simulink model "quad_LQRaccControl_sim"  (R2020a)
settings: Solver=ode4  StartTime=0.0  StopTime=10  FixedStep=0.001  RelTol=1e-3
values from neighbouring files (symbols this model uses):
  L = 0.2    [anim_2Dquad.m]    (also in anim_2Dquad_intercept.m)
undefined symbols (not defined in the file or in its folder): g, I, K, m
settings Model: Creator=Amir  LastModifiedBy=alex
settings DataIOCC: ReturnWorkspaceOutputs=off
settings DebuggingCC: ArithmeticOperatorsInVariantConditions=warning
settings SFSimCC: CustomCodeUndefinedFunction=UseInterfaceOnly

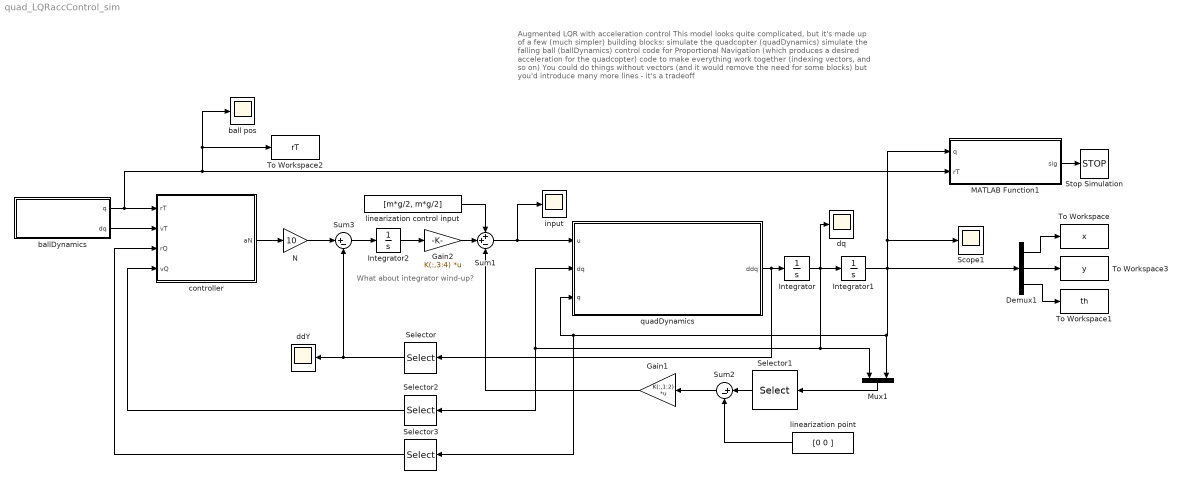
== system quad_LQRaccControl_sim ==
  note: Augmented LQR with acceleration control
      | This model looks quite complicated, but it's made up of a few (much simpler) building blocks:
      |
      | simulate the quadcopter (quadDynamics)
      | simulate the falling ball (ballDynamics)
      | control code for Proportional Navigation (which produces a desired acceleration for the quadcopter)
      | code to make everything work together (indexing vectors, and so on)
      |
      | You could do things without vectors (and it would remove the need for some blocks) but you'd introduce many more lines - it's a tradeoff
  note: What about integrator wind-up?
  Demux1 : Demux  Outputs=3
  Gain1 : Gain  Gain=K(:,1:2)  Multiplication=Matrix(K*u)
  Gain2 : Gain  Gain=K(:,3:4)  Multiplication=Matrix(K*u)
  Integrator : Integrator  InitialCondition=[0 0 0]
  Integrator1 : Integrator  InitialCondition=[0, 0, 0]
  Integrator2 : Integrator
  MATLAB Function1 : MATLAB Function  TreatAsAtomicUnit=on
  Mux1 : Mux  Inputs=2
  N : Gain  Gain=10
  Scope1 : Scope
  Selector : Selector  InputPortWidth=3  IndexOptions=Index vector (dialog)  Indices=[1 2]  OutputSizes=1
  Selector1 : Selector  InputPortWidth=6  IndexOptions=Index vector (dialog)  Indices=[3 6]  OutputSizes=1
  Selector2 : Selector  InputPortWidth=3  IndexOptions=Index vector (dialog)  Indices=[1 2]  OutputSizes=1
  Selector3 : Selector  InputPortWidth=3  IndexOptions=Index vector (dialog)  Indices=[1 2]  OutputSizes=1
  Stop Simulation : Stop
  Sum1 : Sum  Inputs=++-
  Sum2 : Sum  Inputs=|+-
  Sum3 : Sum  Inputs=|+-
  To Workspace : ToWorkspace  VariableName=x  SaveFormat=Structure With Time  SampleTime=0.01
  To Workspace1 : ToWorkspace  VariableName=th  SaveFormat=Structure With Time  SampleTime=0.01
  To Workspace2 : ToWorkspace  VariableName=rT  SaveFormat=Structure With Time  SampleTime=0.01
  To Workspace3 : ToWorkspace  VariableName=y  SaveFormat=Structure With Time  SampleTime=0.01
  ball pos : Scope
  ballDynamics : Subsystem
  controller : MATLAB Function  TreatAsAtomicUnit=on
  ddY : Scope
  dq : Scope
  input : Scope
  linearization control input : Constant  Value=[m*g/2, m*g/2]
  linearization point : Constant  Value=[0 0 ]
  quadDynamics : MATLAB Function  TreatAsAtomicUnit=on
  wires:
  quadDynamics/1(ddq) -> Integrator/1, Selector/1
  Integrator/1 -> Integrator1/1, dq/1, Mux1/1, Selector2/1, quadDynamics/2(dq)
  Sum1/1 -> input/1, quadDynamics/1(u)
  Sum2/1 -> Gain1/1
  linearization point/1 -> Sum2/2
  Integrator1/1 -> Demux1/1, Mux1/2, Selector3/1, quadDynamics/3(q), Scope1/1, MATLAB Function1/1(q)
  Demux1/3 -> To Workspace1/1
  Demux1/1 -> To Workspace/1
  Demux1/2 -> To Workspace3/1
  linearization control input/1 -> Sum1/1
  Gain1/1 -> Sum1/3
  Integrator2/1 -> Gain2/1
  Gain2/1 -> Sum1/2
  Sum3/1 -> Integrator2/1
  Selector/1 -> ddY/1, Sum3/2
  Mux1/1 -> Selector1/1
  Selector1/1 -> Sum2/1
  Selector2/1 -> controller/4(vQ)
  Selector3/1 -> controller/3(rQ)
  controller/1(aN) -> N/1
  N/1 -> Sum3/1
  MATLAB Function1/1(sig) -> Stop Simulation/1
  ballDynamics/1(q) -> MATLAB Function1/2(rT), ball pos/1, To Workspace2/1, controller/1(rT)
  ballDynamics/2(dq) -> controller/2(vT)

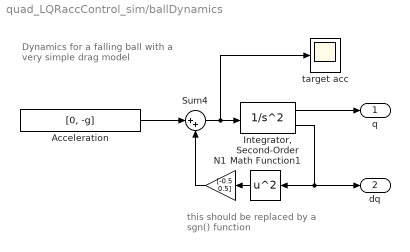
== system quad_LQRaccControl_sim/ballDynamics ==
  note: Dynamics for a falling ball with a very simple drag model
  note: this should be replaced by a sgn() function
  Acceleration : Constant  Value=[0, -g]
  "Integrator, Second-Order" : SecondOrderIntegrator  ICX=[-10 20]  ICDXDT=[15 -1]
  Math Function1 : Math  Operator=square  SignedPower=on  SaturateOnIntegerOverflow=on
  N1 : Gain  Gain=[-0.5 0.5]
  Sum4 : Sum  Inputs=|++
  target acc : Scope
  q : Outport
  dq : Outport  Port=2
  wires:
  Acceleration/1 -> Sum4/1
  N1/1 -> Sum4/2
  "Integrator, Second-Order"/1 -> q/1
  "Integrator, Second-Order"/2 -> dq/1, Math Function1/1
  Math Function1/1 -> N1/1
  Sum4/1 -> target acc/1, "Integrator, Second-Order"/1

== matlab function quad_LQRaccControl_sim/quadDynamics ==
  data: u input; ddq output; dq input; q input; m parameter; I parameter; L parameter; g parameter
function ddq = fullDyn(u,dq,q, m, I, L, g)
%#codegen

%    This function was generated by the Symbolic Math Toolbox version 8.2.
%    23-Apr-2019 00:12:18
% m = 10;
% L = 0.5;
% I = 0.2083; %MOI of a thin rod
% g = 9.81;

F1 = u(1);
F2 = u(2);

x = q(1);
y = q(2);
th = q(3);

dx = dq(1);
dy = dq(2);
dth = dq(3);

t2 = cos(th);
t3 = 1.0./m;
ddq = [-t3.*sin(th).*(F1+F2);t3.*(F1.*t2+F2.*t2-g.*m);(L.*(F1-F2))./(I.*2.0)];

== matlab function quad_LQRaccControl_sim/controller ==
  data: rT input; aN output size=2; vT input; rQ input; vQ input
function aN = pNav(rT, vT, rQ, vQ)
% https://en.wikipedia.org/wiki/Proportional_navigation
% this produces an acceleration which the controller should track
R = rT - rQ;
Rtemp = [R; 0];
Vr = vT - vQ;
Vtemp = [Vr; 0];
omega = cross(Rtemp, Vtemp) / dot(Rtemp, Rtemp);
temp = cross(Vtemp, omega);
aN = temp(1:2);

== matlab function quad_LQRaccControl_sim/MATLAB Function1 ==
  data: q input; sig output; rT input
function sig = collisionCheck(q, rT)

xQ = q(1);
yQ = q(2);

xT = rT(1);
yT = rT(2);

% calculate distances
xDist = abs(xT - xQ);
yDist = abs(yT - yQ);

% if within 1m, assume impact!
if  xDist < 0.1 && yDist < 0.1
    sig = 1;

    % if ball hits the ground
elseif rT(2) < 0
    sig = 1;
    
else
    sig = 0;
end
